simulink library "thermalCoupledCellResolution"  (R2025a)
(part 3 of 3)

  [batteryVoltage22] -> batteryVoltageMux/22
  Module22_outputs/4 -> [numCycles22]
  [numCycles22] -> numCyclesMux/22
  Module22_outputs/5 -> [socCell22]
  [socCell22] -> socCellMux/22
  Module22_outputs/6 -> [socParallelAssembly22]
  [socParallelAssembly22] -> socParallelAssemblyMux/22
  Module22_outputs/7 -> [vParallelAssembly22]
  [vParallelAssembly22] -> vParallelAssemblyMux/22
  Module23_outputs/1 -> [batteryCurrent23]
  [batteryCurrent23] -> batteryCurrentMux/23
  Module23_outputs/2 -> [batteryTemperature23]
  [batteryTemperature23] -> batteryTemperatureMux/23
  Module23_outputs/3 -> [batteryVoltage23]
  [batteryVoltage23] -> batteryVoltageMux/23
  Module23_outputs/4 -> [numCycles23]
  [numCycles23] -> numCyclesMux/23
  Module23_outputs/5 -> [socCell23]
  [socCell23] -> socCellMux/23
  Module23_outputs/6 -> [socParallelAssembly23]
  [socParallelAssembly23] -> socParallelAssemblyMux/23
  Module23_outputs/7 -> [vParallelAssembly23]
  [vParallelAssembly23] -> vParallelAssemblyMux/23
  Module24_outputs/1 -> [batteryCurrent24]
  [batteryCurrent24] -> batteryCurrentMux/24
  Module24_outputs/2 -> [batteryTemperature24]
  [batteryTemperature24] -> batteryTemperatureMux/24
  Module24_outputs/3 -> [batteryVoltage24]
  [batteryVoltage24] -> batteryVoltageMux/24
  Module24_outputs/4 -> [numCycles24]
  [numCycles24] -> numCyclesMux/24
  Module24_outputs/5 -> [socCell24]
  [socCell24] -> socCellMux/24
  Module24_outputs/6 -> [socParallelAssembly24]
  [socParallelAssembly24] -> socParallelAssemblyMux/24
  Module24_outputs/7 -> [vParallelAssembly24]
  [vParallelAssembly24] -> vParallelAssemblyMux/24
  Module25_outputs/1 -> [batteryCurrent25]
  [batteryCurrent25] -> batteryCurrentMux/25
  Module25_outputs/2 -> [batteryTemperature25]
  [batteryTemperature25] -> batteryTemperatureMux/25
  Module25_outputs/3 -> [batteryVoltage25]
  [batteryVoltage25] -> batteryVoltageMux/25
  Module25_outputs/4 -> [numCycles25]
  [numCycles25] -> numCyclesMux/25
  Module25_outputs/5 -> [socCell25]
  [socCell25] -> socCellMux/25
  Module25_outputs/6 -> [socParallelAssembly25]
  [socParallelAssembly25] -> socParallelAssemblyMux/25
  Module25_outputs/7 -> [vParallelAssembly25]
  [vParallelAssembly25] -> vParallelAssemblyMux/25
  Module26_outputs/1 -> [batteryCurrent26]
  [batteryCurrent26] -> batteryCurrentMux/26
  Module26_outputs/2 -> [batteryTemperature26]
  [batteryTemperature26] -> batteryTemperatureMux/26
  Module26_outputs/3 -> [batteryVoltage26]
  [batteryVoltage26] -> batteryVoltageMux/26
  Module26_outputs/4 -> [numCycles26]
  [numCycles26] -> numCyclesMux/26
  Module26_outputs/5 -> [socCell26]
  [socCell26] -> socCellMux/26
  Module26_outputs/6 -> [socParallelAssembly26]
  [socParallelAssembly26] -> socParallelAssemblyMux/26
  Module26_outputs/7 -> [vParallelAssembly26]
  [vParallelAssembly26] -> vParallelAssemblyMux/26
  Module27_outputs/1 -> [batteryCurrent27]
  [batteryCurrent27] -> batteryCurrentMux/27
  Module27_outputs/2 -> [batteryTemperature27]
  [batteryTemperature27] -> batteryTemperatureMux/27
  Module27_outputs/3 -> [batteryVoltage27]
  [batteryVoltage27] -> batteryVoltageMux/27
  Module27_outputs/4 -> [numCycles27]
  [numCycles27] -> numCyclesMux/27
  Module27_outputs/5 -> [socCell27]
  [socCell27] -> socCellMux/27
  Module27_outputs/6 -> [socParallelAssembly27]
  [socParallelAssembly27] -> socParallelAssemblyMux/27
  Module27_outputs/7 -> [vParallelAssembly27]
  [vParallelAssembly27] -> vParallelAssemblyMux/27
  Module28_outputs/1 -> [batteryCurrent28]
  [batteryCurrent28] -> batteryCurrentMux/28
  Module28_outputs/2 -> [batteryTemperature28]
  [batteryTemperature28] -> batteryTemperatureMux/28
  Module28_outputs/3 -> [batteryVoltage28]
  [batteryVoltage28] -> batteryVoltageMux/28
  Module28_outputs/4 -> [numCycles28]
  [numCycles28] -> numCyclesMux/28
  Module28_outputs/5 -> [socCell28]
  [socCell28] -> socCellMux/28
  Module28_outputs/6 -> [socParallelAssembly28]
  [socParallelAssembly28] -> socParallelAssemblyMux/28
  Module28_outputs/7 -> [vParallelAssembly28]
  [vParallelAssembly28] -> vParallelAssemblyMux/28
  Module29_outputs/1 -> [batteryCurrent29]
  [batteryCurrent29] -> batteryCurrentMux/29
  Module29_outputs/2 -> [batteryTemperature29]
  [batteryTemperature29] -> batteryTemperatureMux/29
  Module29_outputs/3 -> [batteryVoltage29]
  [batteryVoltage29] -> batteryVoltageMux/29
  Module29_outputs/4 -> [numCycles29]
  [numCycles29] -> numCyclesMux/29
  Module29_outputs/5 -> [socCell29]
  [socCell29] -> socCellMux/29
  Module29_outputs/6 -> [socParallelAssembly29]
  [socParallelAssembly29] -> socParallelAssemblyMux/29
  Module29_outputs/7 -> [vParallelAssembly29]
  [vParallelAssembly29] -> vParallelAssemblyMux/29
  Module30_outputs/1 -> [batteryCurrent30]
  [batteryCurrent30] -> batteryCurrentMux/30
  Module30_outputs/2 -> [batteryTemperature30]
  [batteryTemperature30] -> batteryTemperatureMux/30
  Module30_outputs/3 -> [batteryVoltage30]
  [batteryVoltage30] -> batteryVoltageMux/30
  Module30_outputs/4 -> [numCycles30]
  [numCycles30] -> numCyclesMux/30
  Module30_outputs/5 -> [socCell30]
  [socCell30] -> socCellMux/30
  Module30_outputs/6 -> [socParallelAssembly30]
  [socParallelAssembly30] -> socParallelAssemblyMux/30
  Module30_outputs/7 -> [vParallelAssembly30]
  [vParallelAssembly30] -> vParallelAssemblyMux/30
  Module31_outputs/1 -> [batteryCurrent31]
  [batteryCurrent31] -> batteryCurrentMux/31
  Module31_outputs/2 -> [batteryTemperature31]
  [batteryTemperature31] -> batteryTemperatureMux/31
  Module31_outputs/3 -> [batteryVoltage31]
  [batteryVoltage31] -> batteryVoltageMux/31
  Module31_outputs/4 -> [numCycles31]
  [numCycles31] -> numCyclesMux/31
  Module31_outputs/5 -> [socCell31]
  [socCell31] -> socCellMux/31
  Module31_outputs/6 -> [socParallelAssembly31]
  [socParallelAssembly31] -> socParallelAssemblyMux/31
  Module31_outputs/7 -> [vParallelAssembly31]
  [vParallelAssembly31] -> vParallelAssemblyMux/31
  Module32_outputs/1 -> [batteryCurrent32]
  [batteryCurrent32] -> batteryCurrentMux/32
  Module32_outputs/2 -> [batteryTemperature32]
  [batteryTemperature32] -> batteryTemperatureMux/32
  Module32_outputs/3 -> [batteryVoltage32]
  [batteryVoltage32] -> batteryVoltageMux/32
  Module32_outputs/4 -> [numCycles32]
  [numCycles32] -> numCyclesMux/32
  Module32_outputs/5 -> [socCell32]
  [socCell32] -> socCellMux/32
  Module32_outputs/6 -> [socParallelAssembly32]
  [socParallelAssembly32] -> socParallelAssemblyMux/32
  Module32_outputs/7 -> [vParallelAssembly32]
  [vParallelAssembly32] -> vParallelAssemblyMux/32
  connections:
  Module02/LConn2 -- Module01/RConn1
  Module03/LConn2 -- Module02/RConn1
  Module04/LConn2 -- Module03/RConn1
  Module05/LConn2 -- Module04/RConn1
  Module06/LConn2 -- Module05/RConn1
  Module07/LConn2 -- Module06/RConn1
  Module08/LConn2 -- Module07/RConn1
  Module09/LConn2 -- Module08/RConn1
  Module10/LConn2 -- Module09/RConn1
  Module11/LConn2 -- Module10/RConn1
  Module12/LConn2 -- Module11/RConn1
  Module13/LConn2 -- Module12/RConn1
  Module14/LConn2 -- Module13/RConn1
  Module15/LConn2 -- Module14/RConn1
  Module16/LConn2 -- Module15/RConn1
  Module17/LConn2 -- Module16/RConn1
  Module18/LConn2 -- Module17/RConn1
  Module19/LConn2 -- Module18/RConn1
  Module20/LConn2 -- Module19/RConn1
  Module21/LConn2 -- Module20/RConn1
  Module22/LConn2 -- Module21/RConn1
  Module23/LConn2 -- Module22/RConn1
  Module24/LConn2 -- Module23/RConn1
  Module25/LConn2 -- Module24/RConn1
  Module26/LConn2 -- Module25/RConn1
  Module27/LConn2 -- Module26/RConn1
  Module28/LConn2 -- Module27/RConn1
  Module29/LConn2 -- Module28/RConn1
  Module30/LConn2 -- Module29/RConn1
  Module31/LConn2 -- Module30/RConn1
  Module32/LConn2 -- Module31/RConn1
  Module01/LConn2 -- +/RConn1
  Module32/RConn1 -- -/RConn1
  AmbH_To_1/LConn1 -- Module01/LConn1
  AmbH_From_1/LConn1 -- AmbH_From_2/LConn1 -- AmbH_From_3/LConn1 -- AmbH_From_4/LConn1 -- AmbH_From_5/LConn1 -- AmbH_From_6/LConn1 -- AmbH_From_7/LConn1 -- AmbH_From_8/LConn1 -- AmbH_From_9/LConn1 -- AmbH_From_10/LConn1 -- AmbH_From_11/LConn1 -- AmbH_From_12/LConn1 -- AmbH_From_13/LConn1 -- AmbH_From_14/LConn1 -- AmbH_From_15/LConn1 -- AmbH_From_16/LConn1 -- AmbH_From_17/LConn1 -- AmbH_From_18/LConn1 -- AmbH_From_19/LConn1 -- AmbH_From_20/LConn1 -- AmbH_From_21/LConn1 -- AmbH_From_22/LConn1 -- AmbH_From_23/LConn1 -- AmbH_From_24/LConn1 -- AmbH_From_25/LConn1 -- AmbH_From_26/LConn1 -- AmbH_From_27/LConn1 -- AmbH_From_28/LConn1 -- AmbH_From_29/LConn1 -- AmbH_From_30/LConn1 -- AmbH_From_31/LConn1 -- AmbH/RConn1 -- AmbH_From_32/LConn1
  AmbH_To_2/LConn1 -- Module02/LConn1
  AmbH_To_3/LConn1 -- Module03/LConn1
  AmbH_To_4/LConn1 -- Module04/LConn1
  AmbH_To_5/LConn1 -- Module05/LConn1
  AmbH_To_6/LConn1 -- Module06/LConn1
  AmbH_To_7/LConn1 -- Module07/LConn1
  AmbH_To_8/LConn1 -- Module08/LConn1
  AmbH_To_9/LConn1 -- Module09/LConn1
  AmbH_To_10/LConn1 -- Module10/LConn1
  AmbH_To_11/LConn1 -- Module11/LConn1
  AmbH_To_12/LConn1 -- Module12/LConn1
  AmbH_To_13/LConn1 -- Module13/LConn1
  AmbH_To_14/LConn1 -- Module14/LConn1
  AmbH_To_15/LConn1 -- Module15/LConn1
  AmbH_To_16/LConn1 -- Module16/LConn1
  AmbH_To_17/LConn1 -- Module17/LConn1
  AmbH_To_18/LConn1 -- Module18/LConn1
  AmbH_To_19/LConn1 -- Module19/LConn1
  AmbH_To_20/LConn1 -- Module20/LConn1
  AmbH_To_21/LConn1 -- Module21/LConn1
  AmbH_To_22/LConn1 -- Module22/LConn1
  AmbH_To_23/LConn1 -- Module23/LConn1
  AmbH_To_24/LConn1 -- Module24/LConn1
  AmbH_To_25/LConn1 -- Module25/LConn1
  AmbH_To_26/LConn1 -- Module26/LConn1
  AmbH_To_27/LConn1 -- Module27/LConn1
  AmbH_To_28/LConn1 -- Module28/LConn1
  AmbH_To_29/LConn1 -- Module29/LConn1
  AmbH_To_30/LConn1 -- Module30/LConn1
  AmbH_To_31/LConn1 -- Module31/LConn1
  AmbH_To_32/LConn1 -- Module32/LConn1
